simulink model "PenduloNoLinealSimulink"  (R2018a)
settings: Solver=ode4  StartTime=0.0  StopTime=10  FixedStep=0.0001  RelTol=1e-3
values from neighbouring files (symbols this model uses):
  b = input('Ingrese un valor para b:')    [ControlOptimno.m]    (also in D_Particiones.m = -w/sin(w*h); D_particiones_a_h.m = -5; ExperimentoInstrumentaacion.m = (sxx*sy-sx*sxy)/(N*sxx-sx*sx); InterpolacionHERMITE.m = 1)
  g = -1    [D_particiones_a_h.m]    (also in InterpolacionHERMITE.m = 1)
  l = (l+1)    (= 2)    [CuadrosMAGICOS.m]    (also in LangrangeF.m = l*((vfx-x(j+1))/(x(i+1)-x(j+1))); Matrix.m = length(A))
  M = length(y)    [ExperimentoInstrumentaacion.m]    (also in Jose.m = rref(M); JoseCarlos.m = rref(M))
  m = 1    [CuadrosMAGICOS.m]    (also in ExperimentoInstrumentaacion.m = (N*sxy-sx*sy)/(N*sxx-sx*sx); InterpolationNewton.m = 2; Jose.m = 2; JoseCarlos.m)
libraries: dspinverses x1
settings Model: Creator=Omie-PC  LastModifiedBy=Benjamin Nicolas

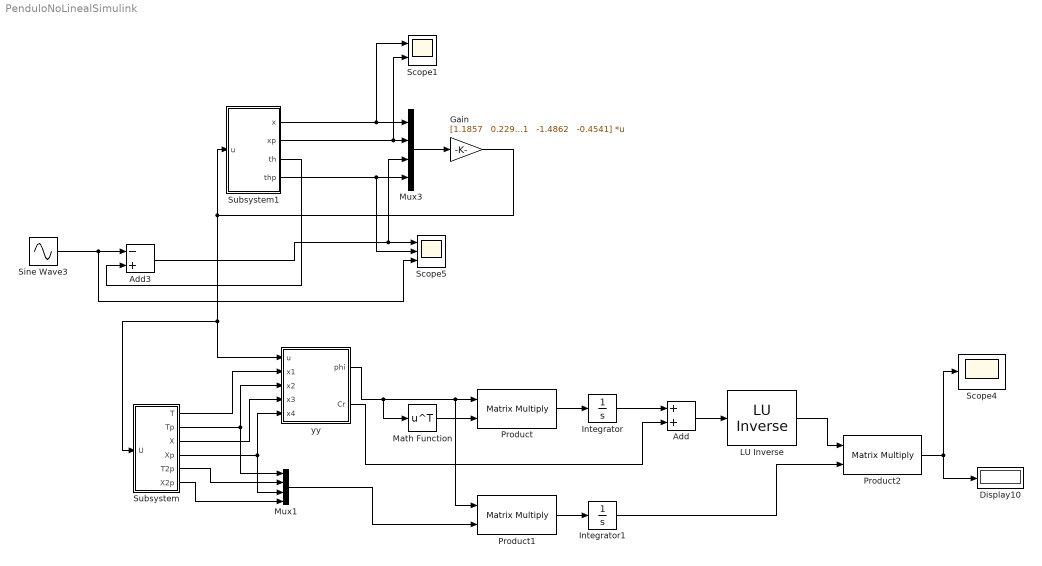
== system PenduloNoLinealSimulink ==
  " LU Inverse" : dspinverses/ LU Inverse
      settings: SourceProductName=DSP System Toolbox
  Add : Sum
  Add3 : Sum  Inputs=-+
  Display10 : Display
  Gain : Gain  Gain="[1.1857   0.2291   -1.4862   -0.4541]"  Multiplication=Matrix(K*u) (u vector)
  Integrator : Integrator
  Integrator1 : Integrator
  Math Function : Math  Operator=transpose  SaturateOnIntegerOverflow=on
  Mux1 : Mux
  Mux3 : Mux
  Product : Product  Multiplication=Matrix(*)
  Product1 : Product  Multiplication=Matrix(*)
  Product2 : Product  Multiplication=Matrix(*)
  Scope1 : Scope  NumInputPorts=2
  Scope4 : Scope
  Scope5 : Scope  NumInputPorts=3
  Sine Wave3 : Sin  Amplitude=0.5  Frequency=10  SampleTime=0
  Subsystem : Subsystem
  Subsystem1 : Subsystem
  yy : MATLAB Function  TreatAsAtomicUnit=on
  wires:
  yy/2(Cr) -> Add/2
  Product/1 -> Integrator/1
  Product1/1 -> Integrator1/1
  " LU Inverse"/1 -> Product2/1
  yy/1(phi) -> Product1/1, Product/1, Math Function/1
  Integrator1/1 -> Product2/2
  Mux1/1 -> Product1/2
  Add/1 -> " LU Inverse"/1
  Math Function/1 -> Product/2
  Integrator/1 -> Add/1
  Subsystem/1(T) -> yy/2(x1)
  Subsystem/2(Tp) -> Mux1/1, yy/3(x2)
  Subsystem/3(X) -> yy/4(x3)
  Subsystem/4(Xp) -> Mux1/3, yy/5(x4)
  Subsystem/5(T2p) -> Mux1/2
  Subsystem/6(X2p) -> Mux1/4
  Product2/1 -> Scope4/1, Display10/1
  Add3/1 -> Mux3/3, Scope5/1
  Subsystem1/1(x) -> Scope1/1, Mux3/1
  Gain/1 -> Subsystem1/1(u), Subsystem/1(U), yy/1(u)
  Mux3/1 -> Gain/1
  Subsystem1/2(xp) -> Scope1/2, Mux3/2
  Subsystem1/3(th) -> Add3/2
  Subsystem1/4(thp) -> Scope5/2, Mux3/4
  Sine Wave3/1 -> Scope5/3, Add3/1

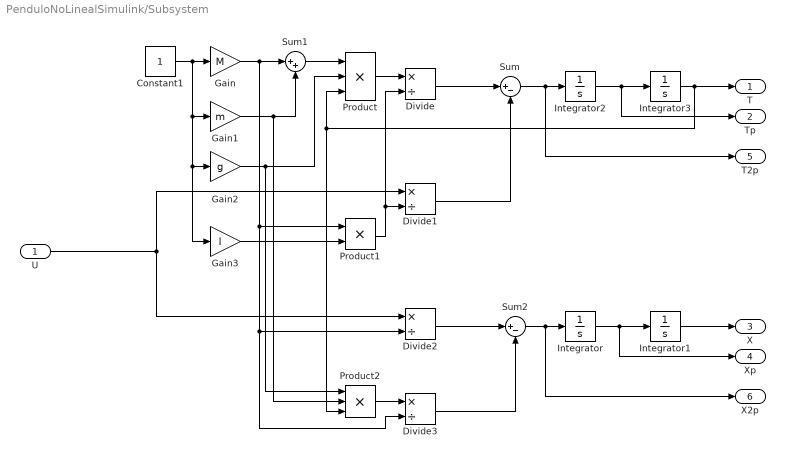
== system PenduloNoLinealSimulink/Subsystem ==
  U : Inport
  Constant1 : Constant
  Divide{,1..3} (4 alike) : Product  Inputs=*/
  Gain : Gain  Gain=M
  Gain1 : Gain  Gain=m
  Gain2 : Gain  Gain=g
  Gain3 : Gain  Gain=l
  Integrator : Integrator
  Integrator1 : Integrator  InitialCondition=0.1
  Integrator2 : Integrator  InitialCondition=0.01
  Integrator3 : Integrator  InitialCondition=0.1
  Product : Product  Inputs=3
  Product1 : Product
  Product2 : Product  Inputs=3
  Sum : Sum  Inputs=|+-
  Sum1 : Sum  Inputs=|++
  Sum2 : Sum  Inputs=|+-
  T : Outport
  Tp : Outport  Port=2
  X : Outport  Port=3
  Xp : Outport  Port=4
  T2p : Outport  Port=5
  X2p : Outport  Port=6
  wires:
  Divide1/1 -> Sum/2
  Gain/1 -> Divide3/2, Divide2/2, Product1/1, Sum1/1
  Divide/1 -> Sum/1
  Gain1/1 -> Product2/2, Sum1/2
  U/1 -> Divide1/1, Divide2/1
  Constant1/1 -> Gain3/1, Gain2/1, Gain1/1, Gain/1
  Integrator/1 -> Xp/1, Integrator1/1
  Divide3/1 -> Sum2/2
  Integrator2/1 -> Tp/1, Integrator3/1
  Gain2/1 -> Product2/1, Product/2
  Integrator3/1 -> T/1, Product/3, Product2/3
  Product1/1 -> Divide/2, Divide1/2
  Product2/1 -> Divide3/1
  Integrator1/1 -> X/1
  Product/1 -> Divide/1
  Sum1/1 -> Product/1
  Divide2/1 -> Sum2/1
  Sum/1 -> T2p/1, Integrator2/1
  Gain3/1 -> Product1/2
  Sum2/1 -> X2p/1, Integrator/1

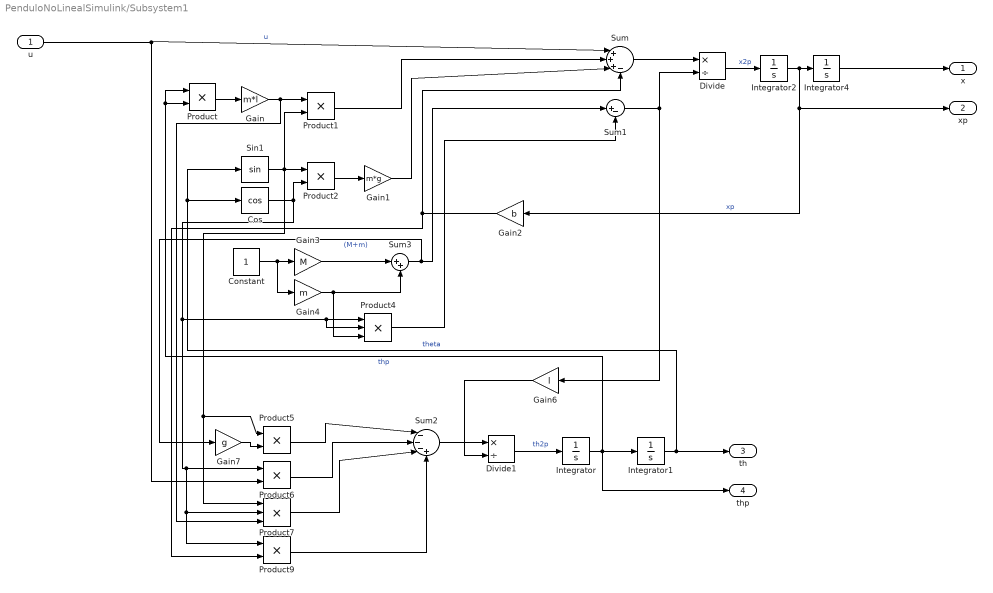
== system PenduloNoLinealSimulink/Subsystem1 ==
  u : Inport
  Constant : Constant
  Cos : Trigonometry  Operator=cos
  Divide : Product  Inputs=*/
  Divide1 : Product  Inputs=*/
  Gain : Gain  Gain=m*l
  Gain1 : Gain  Gain=m*g
  Gain2 : Gain  Gain=b
  Gain3 : Gain  Gain=M
  Gain4 : Gain  Gain=m
  Gain6 : Gain  Gain=l
  Gain7 : Gain  Gain=g
  Integrator{,1..2,4} (4 alike) : Integrator  InitialCondition=pi/4
  Product{,1..2,5..6,9} (6 alike) : Product
  Product4 : Product  Inputs=3
  Product7 : Product  Inputs=3
  Sin1 : Trigonometry
  Sum : Sum  Inputs=|+++-
  Sum1 : Sum  Inputs=|+-
  Sum2 : Sum  Inputs=|---+
  Sum3 : Sum  Inputs=|++
  x : Outport
  xp : Outport  Port=2
  th : Outport  Port=3
  thp : Outport  Port=4
  wires:
  Gain/1 -> Product7/3, Product1/1
  Divide/1 -> Integrator2/1  "x2p"
  Sum/1 -> Divide/1
  Integrator/1 -> Product/2, Product/1, thp/1, Integrator1/1  "thp"
  Product7/1 -> Sum2/3
  Gain6/1 -> Divide1/2
  Product6/1 -> Sum2/2
  Gain7/1 -> Product5/2
  Gain4/1 -> Product4/3, Sum3/2
  Product5/1 -> Sum2/1
  Product9/1 -> Sum2/4
  Sum2/1 -> Divide1/1
  Product/1 -> Gain/1
  Sum3/1 -> Gain7/1, Sum1/1  "(M+m)"
  Gain2/1 -> Product9/2, Sum/4
  Divide1/1 -> Integrator/1  "th2p"
  Sum1/1 -> Gain6/1, Divide/2
  Integrator4/1 -> x/1
  u/1 -> Sum/1, Product6/2  "u"
  Sin1/1 -> Product1/2, Product7/1, Product5/1, Product2/1
  Constant/1 -> Gain4/1, Gain3/1
  Product1/1 -> Sum/2
  Gain3/1 -> Sum3/1
  Integrator1/1 -> Sin1/1, Cos/1, th/1  "theta"
  Cos/1 -> Product9/1, Product7/2, Product6/1, Product4/2, Product4/1, Product2/2
  Product4/1 -> Sum1/2
  Integrator2/1 -> Gain2/1, xp/1, Integrator4/1  "xp"
  Gain1/1 -> Sum/3
  Product2/1 -> Gain1/1

== matlab function PenduloNoLinealSimulink/yy ==
  data: u input; x1 input; phi output; x2 input; x3 input; Cr output; x4 input
function [phi,Cr]  = fcn(u,x1,x2,x3,x4)
k=0.1;
Cr=k*eye(6);
% phi = [x2,0,0,0;0,sin(x1)/cos(x1)^2,0,0;0,u,/cos(x1),0,0;0,x2^2*sin(x1)/cos(x1),0,0;0,x4/cos(x1),0,0;0,0,1,0;0,0,0,u/cos(x1)^2;0,0,0,x2^2*sin(x1)/cos(x1)^2;0,0,0,sin(x1)/cos(x1);0,0,0,x4/cos(x1)^2];
ph = [0,0,0,0,x2,0;x1,u,0,0,0,0;0,0,0,0,0,x4;0,0,u,x1,0,0];
phi=ph'
